simulink model "w3_warplab_trigger_proc"  (Simulink 7.7)
settings: Solver=ode45  StartTime=0.0  StopTime=60  RelTol=1e-3
InitFcn:
  | w3_warplab_trigger_proc_init
StartFcn:
  | w3_warplab_trigger_proc_init
undefined symbols (not defined in the file): gcbh, xlBlockLoadCallback, xlGetNormalizedPeriod
libraries: xbsIndex_r4 x1289, xbsEDKLib_r4 x1, simulink x1
(part 6 of 10)

== system w3_warplab_trigger_proc/Registers/Input Configuration Slice7 ==
  32b : Inport
  b30 : xbsIndex_r4/Slice  nbits=1  boolean_output=off  mode=Lower Bit Location + Width  bit1=0  base1=MSB of Input  bit0=30  base0=LSB of Input  dbl_ovrd=off  block_type=slice
  b31 : xbsIndex_r4/Slice  nbits=1  boolean_output=off  mode=Lower Bit Location + Width  bit1=0  base1=MSB of Input  bit0=31  base0=LSB of Input  dbl_ovrd=off  block_type=slice
  b[0:4] : xbsIndex_r4/Slice  nbits=5  boolean_output=off  mode=Lower Bit Location + Width  bit1=0  base1=MSB of Input  bit0=0  base0=LSB of Input  dbl_ovrd=off  block_type=slice
  Delay : Outport
  Debounce : Outport  Port=2
  Disable : Outport  Port=3
  wires:
  b31/1 -> Disable/1
  b30/1 -> Debounce/1
  b[0:4]/1 -> Delay/1
  32b/1 -> b[0:4]/1, b30/1, b31/1

== system w3_warplab_trigger_proc/Registers/Input Configuration Slice8 ==
  32b : Inport
  b29 : xbsIndex_r4/Slice  nbits=1  boolean_output=off  mode=Lower Bit Location + Width  bit1=0  base1=MSB of Input  bit0=29  base0=LSB of Input  dbl_ovrd=off  block_type=slice
  b30 : xbsIndex_r4/Slice  nbits=1  boolean_output=off  mode=Lower Bit Location + Width  bit1=0  base1=MSB of Input  bit0=30  base0=LSB of Input  dbl_ovrd=off  block_type=slice
  b31 : xbsIndex_r4/Slice  nbits=1  boolean_output=off  mode=Lower Bit Location + Width  bit1=0  base1=MSB of Input  bit0=31  base0=LSB of Input  dbl_ovrd=off  block_type=slice
  b[0:4] : xbsIndex_r4/Slice  nbits=5  boolean_output=off  mode=Lower Bit Location + Width  bit1=0  base1=MSB of Input  bit0=0  base0=LSB of Input  dbl_ovrd=off  block_type=slice
  Delay : Outport
  HW_SW_Sel : Outport  Port=2
  Debounce : Outport  Port=3
  Disable : Outport  Port=4
  wires:
  b31/1 -> Disable/1
  b30/1 -> Debounce/1
  b[0:4]/1 -> Delay/1
  32b/1 -> b[0:4]/1, b30/1, b31/1, b29/1
  b29/1 -> HW_SW_Sel/1

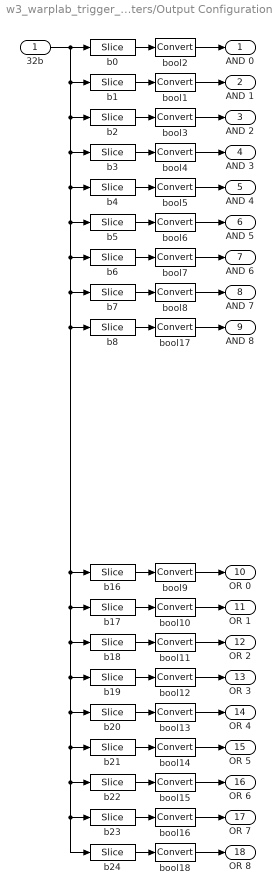
== system w3_warplab_trigger_proc/Registers/Output Configuration Slice ==
  32b : Inport
  b0 : xbsIndex_r4/Slice  nbits=1  boolean_output=off  mode=Lower Bit Location + Width  bit1=0  base1=MSB of Input  bit0=0  base0=LSB of Input  dbl_ovrd=off  block_type=slice
  b1 : xbsIndex_r4/Slice  nbits=1  boolean_output=off  mode=Lower Bit Location + Width  bit1=0  base1=MSB of Input  bit0=1  base0=LSB of Input  dbl_ovrd=off  block_type=slice
  b16 : xbsIndex_r4/Slice  nbits=1  boolean_output=off  mode=Lower Bit Location + Width  bit1=0  base1=MSB of Input  bit0=16  base0=LSB of Input  dbl_ovrd=off  block_type=slice
  b17 : xbsIndex_r4/Slice  nbits=1  boolean_output=off  mode=Lower Bit Location + Width  bit1=0  base1=MSB of Input  bit0=17  base0=LSB of Input  dbl_ovrd=off  block_type=slice
  b18 : xbsIndex_r4/Slice  nbits=1  boolean_output=off  mode=Lower Bit Location + Width  bit1=0  base1=MSB of Input  bit0=18  base0=LSB of Input  dbl_ovrd=off  block_type=slice
  b19 : xbsIndex_r4/Slice  nbits=1  boolean_output=off  mode=Lower Bit Location + Width  bit1=0  base1=MSB of Input  bit0=19  base0=LSB of Input  dbl_ovrd=off  block_type=slice
  b2 : xbsIndex_r4/Slice  nbits=1  boolean_output=off  mode=Lower Bit Location + Width  bit1=0  base1=MSB of Input  bit0=2  base0=LSB of Input  dbl_ovrd=off  block_type=slice
  b20 : xbsIndex_r4/Slice  nbits=1  boolean_output=off  mode=Lower Bit Location + Width  bit1=0  base1=MSB of Input  bit0=20  base0=LSB of Input  dbl_ovrd=off  block_type=slice
  b21 : xbsIndex_r4/Slice  nbits=1  boolean_output=off  mode=Lower Bit Location + Width  bit1=0  base1=MSB of Input  bit0=21  base0=LSB of Input  dbl_ovrd=off  block_type=slice
  b22 : xbsIndex_r4/Slice  nbits=1  boolean_output=off  mode=Lower Bit Location + Width  bit1=0  base1=MSB of Input  bit0=22  base0=LSB of Input  dbl_ovrd=off  block_type=slice
  b23 : xbsIndex_r4/Slice  nbits=1  boolean_output=off  mode=Lower Bit Location + Width  bit1=0  base1=MSB of Input  bit0=23  base0=LSB of Input  dbl_ovrd=off  block_type=slice
  b24 : xbsIndex_r4/Slice  nbits=1  boolean_output=off  mode=Lower Bit Location + Width  bit1=0  base1=MSB of Input  bit0=24  base0=LSB of Input  dbl_ovrd=off  block_type=slice
  b3 : xbsIndex_r4/Slice  nbits=1  boolean_output=off  mode=Lower Bit Location + Width  bit1=0  base1=MSB of Input  bit0=3  base0=LSB of Input  dbl_ovrd=off  block_type=slice
  b4 : xbsIndex_r4/Slice  nbits=1  boolean_output=off  mode=Lower Bit Location + Width  bit1=0  base1=MSB of Input  bit0=4  base0=LSB of Input  dbl_ovrd=off  block_type=slice
  b5 : xbsIndex_r4/Slice  nbits=1  boolean_output=off  mode=Lower Bit Location + Width  bit1=0  base1=MSB of Input  bit0=5  base0=LSB of Input  dbl_ovrd=off  block_type=slice
  b6 : xbsIndex_r4/Slice  nbits=1  boolean_output=off  mode=Lower Bit Location + Width  bit1=0  base1=MSB of Input  bit0=6  base0=LSB of Input  dbl_ovrd=off  block_type=slice
  b7 : xbsIndex_r4/Slice  nbits=1  boolean_output=off  mode=Lower Bit Location + Width  bit1=0  base1=MSB of Input  bit0=7  base0=LSB of Input  dbl_ovrd=off  block_type=slice
  b8 : xbsIndex_r4/Slice  nbits=1  boolean_output=off  mode=Lower Bit Location + Width  bit1=0  base1=MSB of Input  bit0=8  base0=LSB of Input  dbl_ovrd=off  block_type=slice
  bool{1..18} (18 alike) : xbsIndex_r4/Convert  gui_display_data_type=Boolean  arith_type=Boolean  n_bits=16  bin_pt=14  float_type=Single  exp_bits=8  fraction_bits=24  quantization=Truncate  overflow=Wrap  en=off  latency=0  dbl_ovrd=off  pipeline=off  block_type=convert
  AND 0 : Outport
  AND 1 : Outport  Port=2
  AND 2 : Outport  Port=3
  AND 3 : Outport  Port=4
  AND 4 : Outport  Port=5
  AND 5 : Outport  Port=6
  AND 6 : Outport  Port=7
  AND 7 : Outport  Port=8
  AND 8 : Outport  Port=9
  OR 0 : Outport  Port=10
  OR 1 : Outport  Port=11
  OR 2 : Outport  Port=12
  OR 3 : Outport  Port=13
  OR 4 : Outport  Port=14
  OR 5 : Outport  Port=15
  OR 6 : Outport  Port=16
  OR 7 : Outport  Port=17
  OR 8 : Outport  Port=18
  wires:
  32b/1 -> b0/1, b1/1, b2/1, b3/1, b4/1, b5/1, b6/1, b7/1, b16/1, b17/1, b18/1, b19/1, b20/1, b21/1, b22/1, b23/1, b24/1, b8/1
  b0/1 -> bool2/1
  b1/1 -> bool1/1
  b2/1 -> bool3/1
  b3/1 -> bool4/1
  b4/1 -> bool5/1
  b5/1 -> bool6/1
  b6/1 -> bool7/1
  b7/1 -> bool8/1
  b16/1 -> bool9/1
  b17/1 -> bool10/1
  b18/1 -> bool11/1
  b19/1 -> bool12/1
  b20/1 -> bool13/1
  b21/1 -> bool14/1
  b22/1 -> bool15/1
  b23/1 -> bool16/1
  bool2/1 -> AND 0/1
  bool1/1 -> AND 1/1
  bool3/1 -> AND 2/1
  bool4/1 -> AND 3/1
  bool5/1 -> AND 4/1
  bool6/1 -> AND 5/1
  bool7/1 -> AND 6/1
  bool8/1 -> AND 7/1
  bool9/1 -> OR 0/1
  bool10/1 -> OR 1/1
  bool11/1 -> OR 2/1
  bool12/1 -> OR 3/1
  bool13/1 -> OR 4/1
  bool14/1 -> OR 5/1
  bool15/1 -> OR 6/1
  bool16/1 -> OR 7/1
  b8/1 -> bool17/1
  bool17/1 -> AND 8/1
  b24/1 -> bool18/1
  bool18/1 -> OR 8/1

== system w3_warplab_trigger_proc/Registers/Output Configuration Slice1 ==
  32b : Inport
  b30 : xbsIndex_r4/Slice  nbits=1  boolean_output=off  mode=Lower Bit Location + Width  bit1=0  base1=MSB of Input  bit0=30  base0=LSB of Input  dbl_ovrd=off  block_type=slice
  b31 : xbsIndex_r4/Slice  nbits=1  boolean_output=off  mode=Lower Bit Location + Width  bit1=0  base1=MSB of Input  bit0=31  base0=LSB of Input  dbl_ovrd=off  block_type=slice
  b[0:15] : xbsIndex_r4/Slice  nbits=16  boolean_output=off  mode=Lower Bit Location + Width  bit1=0  base1=MSB of Input  bit0=0  base0=LSB of Input  dbl_ovrd=off  block_type=slice
  bool1 : xbsIndex_r4/Convert  gui_display_data_type=Boolean  arith_type=Boolean  n_bits=16  bin_pt=14  float_type=Single  exp_bits=8  fraction_bits=24  quantization=Truncate  overflow=Wrap  en=off  latency=0  dbl_ovrd=off  pipeline=off  block_type=convert
  bool17 : xbsIndex_r4/Convert  gui_display_data_type=Boolean  arith_type=Boolean  n_bits=16  bin_pt=14  float_type=Single  exp_bits=8  fraction_bits=24  quantization=Truncate  overflow=Wrap  en=off  latency=0  dbl_ovrd=off  pipeline=off  block_type=convert
  DELAY : Outport
  BYPASS : Outport  Port=2
  DISABLE : Outport  Port=3
  wires:
  32b/1 -> b[0:15]/1, b31/1, b30/1
  b31/1 -> bool17/1
  bool17/1 -> DISABLE/1
  b[0:15]/1 -> DELAY/1
  b30/1 -> bool1/1
  bool1/1 -> BYPASS/1

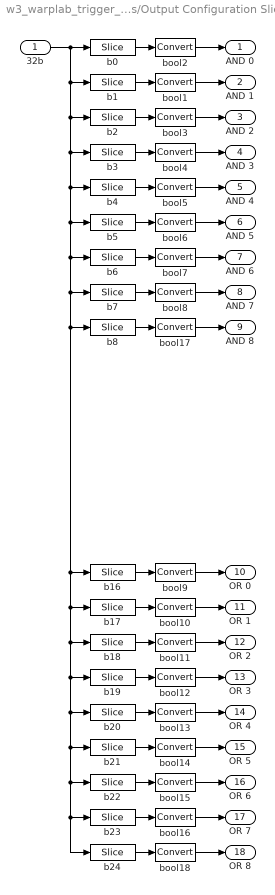
== system w3_warplab_trigger_proc/Registers/Output Configuration Slice12 ==
  32b : Inport
  b0 : xbsIndex_r4/Slice  nbits=1  boolean_output=off  mode=Lower Bit Location + Width  bit1=0  base1=MSB of Input  bit0=0  base0=LSB of Input  dbl_ovrd=off  block_type=slice
  b1 : xbsIndex_r4/Slice  nbits=1  boolean_output=off  mode=Lower Bit Location + Width  bit1=0  base1=MSB of Input  bit0=1  base0=LSB of Input  dbl_ovrd=off  block_type=slice
  b16 : xbsIndex_r4/Slice  nbits=1  boolean_output=off  mode=Lower Bit Location + Width  bit1=0  base1=MSB of Input  bit0=16  base0=LSB of Input  dbl_ovrd=off  block_type=slice
  b17 : xbsIndex_r4/Slice  nbits=1  boolean_output=off  mode=Lower Bit Location + Width  bit1=0  base1=MSB of Input  bit0=17  base0=LSB of Input  dbl_ovrd=off  block_type=slice
  b18 : xbsIndex_r4/Slice  nbits=1  boolean_output=off  mode=Lower Bit Location + Width  bit1=0  base1=MSB of Input  bit0=18  base0=LSB of Input  dbl_ovrd=off  block_type=slice
  b19 : xbsIndex_r4/Slice  nbits=1  boolean_output=off  mode=Lower Bit Location + Width  bit1=0  base1=MSB of Input  bit0=19  base0=LSB of Input  dbl_ovrd=off  block_type=slice
  b2 : xbsIndex_r4/Slice  nbits=1  boolean_output=off  mode=Lower Bit Location + Width  bit1=0  base1=MSB of Input  bit0=2  base0=LSB of Input  dbl_ovrd=off  block_type=slice
  b20 : xbsIndex_r4/Slice  nbits=1  boolean_output=off  mode=Lower Bit Location + Width  bit1=0  base1=MSB of Input  bit0=20  base0=LSB of Input  dbl_ovrd=off  block_type=slice
  b21 : xbsIndex_r4/Slice  nbits=1  boolean_output=off  mode=Lower Bit Location + Width  bit1=0  base1=MSB of Input  bit0=21  base0=LSB of Input  dbl_ovrd=off  block_type=slice
  b22 : xbsIndex_r4/Slice  nbits=1  boolean_output=off  mode=Lower Bit Location + Width  bit1=0  base1=MSB of Input  bit0=22  base0=LSB of Input  dbl_ovrd=off  block_type=slice
  b23 : xbsIndex_r4/Slice  nbits=1  boolean_output=off  mode=Lower Bit Location + Width  bit1=0  base1=MSB of Input  bit0=23  base0=LSB of Input  dbl_ovrd=off  block_type=slice
  b24 : xbsIndex_r4/Slice  nbits=1  boolean_output=off  mode=Lower Bit Location + Width  bit1=0  base1=MSB of Input  bit0=24  base0=LSB of Input  dbl_ovrd=off  block_type=slice
  b3 : xbsIndex_r4/Slice  nbits=1  boolean_output=off  mode=Lower Bit Location + Width  bit1=0  base1=MSB of Input  bit0=3  base0=LSB of Input  dbl_ovrd=off  block_type=slice
  b4 : xbsIndex_r4/Slice  nbits=1  boolean_output=off  mode=Lower Bit Location + Width  bit1=0  base1=MSB of Input  bit0=4  base0=LSB of Input  dbl_ovrd=off  block_type=slice
  b5 : xbsIndex_r4/Slice  nbits=1  boolean_output=off  mode=Lower Bit Location + Width  bit1=0  base1=MSB of Input  bit0=5  base0=LSB of Input  dbl_ovrd=off  block_type=slice
  b6 : xbsIndex_r4/Slice  nbits=1  boolean_output=off  mode=Lower Bit Location + Width  bit1=0  base1=MSB of Input  bit0=6  base0=LSB of Input  dbl_ovrd=off  block_type=slice
  b7 : xbsIndex_r4/Slice  nbits=1  boolean_output=off  mode=Lower Bit Location + Width  bit1=0  base1=MSB of Input  bit0=7  base0=LSB of Input  dbl_ovrd=off  block_type=slice
  b8 : xbsIndex_r4/Slice  nbits=1  boolean_output=off  mode=Lower Bit Location + Width  bit1=0  base1=MSB of Input  bit0=8  base0=LSB of Input  dbl_ovrd=off  block_type=slice
  bool{1..18} (18 alike) : xbsIndex_r4/Convert  gui_display_data_type=Boolean  arith_type=Boolean  n_bits=16  bin_pt=14  float_type=Single  exp_bits=8  fraction_bits=24  quantization=Truncate  overflow=Wrap  en=off  latency=0  dbl_ovrd=off  pipeline=off  block_type=convert
  AND 0 : Outport
  AND 1 : Outport  Port=2
  AND 2 : Outport  Port=3
  AND 3 : Outport  Port=4
  AND 4 : Outport  Port=5
  AND 5 : Outport  Port=6
  AND 6 : Outport  Port=7
  AND 7 : Outport  Port=8
  AND 8 : Outport  Port=9
  OR 0 : Outport  Port=10
  OR 1 : Outport  Port=11
  OR 2 : Outport  Port=12
  OR 3 : Outport  Port=13
  OR 4 : Outport  Port=14
  OR 5 : Outport  Port=15
  OR 6 : Outport  Port=16
  OR 7 : Outport  Port=17
  OR 8 : Outport  Port=18
  wires:
  32b/1 -> b0/1, b1/1, b2/1, b3/1, b4/1, b5/1, b6/1, b7/1, b16/1, b17/1, b18/1, b19/1, b20/1, b21/1, b22/1, b23/1, b24/1, b8/1
  b0/1 -> bool2/1
  b1/1 -> bool1/1
  b2/1 -> bool3/1
  b3/1 -> bool4/1
  b4/1 -> bool5/1
  b5/1 -> bool6/1
  b6/1 -> bool7/1
  b7/1 -> bool8/1
  b16/1 -> bool9/1
  b17/1 -> bool10/1
  b18/1 -> bool11/1
  b19/1 -> bool12/1
  b20/1 -> bool13/1
  b21/1 -> bool14/1
  b22/1 -> bool15/1
  b23/1 -> bool16/1
  bool2/1 -> AND 0/1
  bool1/1 -> AND 1/1
  bool3/1 -> AND 2/1
  bool4/1 -> AND 3/1
  bool5/1 -> AND 4/1
  bool6/1 -> AND 5/1
  bool7/1 -> AND 6/1
  bool8/1 -> AND 7/1
  bool9/1 -> OR 0/1
  bool10/1 -> OR 1/1
  bool11/1 -> OR 2/1
  bool12/1 -> OR 3/1
  bool13/1 -> OR 4/1
  bool14/1 -> OR 5/1
  bool15/1 -> OR 6/1
  bool16/1 -> OR 7/1
  b8/1 -> bool17/1
  bool17/1 -> AND 8/1
  b24/1 -> bool18/1
  bool18/1 -> OR 8/1

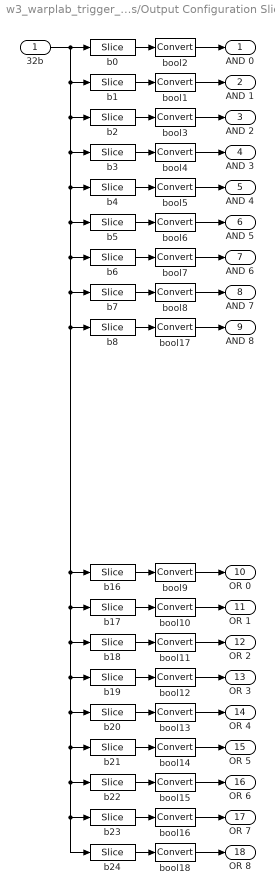
== system w3_warplab_trigger_proc/Registers/Output Configuration Slice14 ==
  32b : Inport
  b0 : xbsIndex_r4/Slice  nbits=1  boolean_output=off  mode=Lower Bit Location + Width  bit1=0  base1=MSB of Input  bit0=0  base0=LSB of Input  dbl_ovrd=off  block_type=slice
  b1 : xbsIndex_r4/Slice  nbits=1  boolean_output=off  mode=Lower Bit Location + Width  bit1=0  base1=MSB of Input  bit0=1  base0=LSB of Input  dbl_ovrd=off  block_type=slice
  b16 : xbsIndex_r4/Slice  nbits=1  boolean_output=off  mode=Lower Bit Location + Width  bit1=0  base1=MSB of Input  bit0=16  base0=LSB of Input  dbl_ovrd=off  block_type=slice
  b17 : xbsIndex_r4/Slice  nbits=1  boolean_output=off  mode=Lower Bit Location + Width  bit1=0  base1=MSB of Input  bit0=17  base0=LSB of Input  dbl_ovrd=off  block_type=slice
  b18 : xbsIndex_r4/Slice  nbits=1  boolean_output=off  mode=Lower Bit Location + Width  bit1=0  base1=MSB of Input  bit0=18  base0=LSB of Input  dbl_ovrd=off  block_type=slice
  b19 : xbsIndex_r4/Slice  nbits=1  boolean_output=off  mode=Lower Bit Location + Width  bit1=0  base1=MSB of Input  bit0=19  base0=LSB of Input  dbl_ovrd=off  block_type=slice
  b2 : xbsIndex_r4/Slice  nbits=1  boolean_output=off  mode=Lower Bit Location + Width  bit1=0  base1=MSB of Input  bit0=2  base0=LSB of Input  dbl_ovrd=off  block_type=slice
  b20 : xbsIndex_r4/Slice  nbits=1  boolean_output=off  mode=Lower Bit Location + Width  bit1=0  base1=MSB of Input  bit0=20  base0=LSB of Input  dbl_ovrd=off  block_type=slice
  b21 : xbsIndex_r4/Slice  nbits=1  boolean_output=off  mode=Lower Bit Location + Width  bit1=0  base1=MSB of Input  bit0=21  base0=LSB of Input  dbl_ovrd=off  block_type=slice
  b22 : xbsIndex_r4/Slice  nbits=1  boolean_output=off  mode=Lower Bit Location + Width  bit1=0  base1=MSB of Input  bit0=22  base0=LSB of Input  dbl_ovrd=off  block_type=slice
  b23 : xbsIndex_r4/Slice  nbits=1  boolean_output=off  mode=Lower Bit Location + Width  bit1=0  base1=MSB of Input  bit0=23  base0=LSB of Input  dbl_ovrd=off  block_type=slice
  b24 : xbsIndex_r4/Slice  nbits=1  boolean_output=off  mode=Lower Bit Location + Width  bit1=0  base1=MSB of Input  bit0=24  base0=LSB of Input  dbl_ovrd=off  block_type=slice
  b3 : xbsIndex_r4/Slice  nbits=1  boolean_output=off  mode=Lower Bit Location + Width  bit1=0  base1=MSB of Input  bit0=3  base0=LSB of Input  dbl_ovrd=off  block_type=slice
  b4 : xbsIndex_r4/Slice  nbits=1  boolean_output=off  mode=Lower Bit Location + Width  bit1=0  base1=MSB of Input  bit0=4  base0=LSB of Input  dbl_ovrd=off  block_type=slice
  b5 : xbsIndex_r4/Slice  nbits=1  boolean_output=off  mode=Lower Bit Location + Width  bit1=0  base1=MSB of Input  bit0=5  base0=LSB of Input  dbl_ovrd=off  block_type=slice
  b6 : xbsIndex_r4/Slice  nbits=1  boolean_output=off  mode=Lower Bit Location + Width  bit1=0  base1=MSB of Input  bit0=6  base0=LSB of Input  dbl_ovrd=off  block_type=slice
  b7 : xbsIndex_r4/Slice  nbits=1  boolean_output=off  mode=Lower Bit Location + Width  bit1=0  base1=MSB of Input  bit0=7  base0=LSB of Input  dbl_ovrd=off  block_type=slice
  b8 : xbsIndex_r4/Slice  nbits=1  boolean_output=off  mode=Lower Bit Location + Width  bit1=0  base1=MSB of Input  bit0=8  base0=LSB of Input  dbl_ovrd=off  block_type=slice
  bool{1..18} (18 alike) : xbsIndex_r4/Convert  gui_display_data_type=Boolean  arith_type=Boolean  n_bits=16  bin_pt=14  float_type=Single  exp_bits=8  fraction_bits=24  quantization=Truncate  overflow=Wrap  en=off  latency=0  dbl_ovrd=off  pipeline=off  block_type=convert
  AND 0 : Outport
  AND 1 : Outport  Port=2
  AND 2 : Outport  Port=3
  AND 3 : Outport  Port=4
  AND 4 : Outport  Port=5
  AND 5 : Outport  Port=6
  AND 6 : Outport  Port=7
  AND 7 : Outport  Port=8
  AND 8 : Outport  Port=9
  OR 0 : Outport  Port=10
  OR 1 : Outport  Port=11
  OR 2 : Outport  Port=12
  OR 3 : Outport  Port=13
  OR 4 : Outport  Port=14
  OR 5 : Outport  Port=15
  OR 6 : Outport  Port=16
  OR 7 : Outport  Port=17
  OR 8 : Outport  Port=18
  wires:
  32b/1 -> b0/1, b1/1, b2/1, b3/1, b4/1, b5/1, b6/1, b7/1, b16/1, b17/1, b18/1, b19/1, b20/1, b21/1, b22/1, b23/1, b24/1, b8/1
  b0/1 -> bool2/1
  b1/1 -> bool1/1
  b2/1 -> bool3/1
  b3/1 -> bool4/1
  b4/1 -> bool5/1
  b5/1 -> bool6/1
  b6/1 -> bool7/1
  b7/1 -> bool8/1
  b16/1 -> bool9/1
  b17/1 -> bool10/1
  b18/1 -> bool11/1
  b19/1 -> bool12/1
  b20/1 -> bool13/1
  b21/1 -> bool14/1
  b22/1 -> bool15/1
  b23/1 -> bool16/1
  bool2/1 -> AND 0/1
  bool1/1 -> AND 1/1
  bool3/1 -> AND 2/1
  bool4/1 -> AND 3/1
  bool5/1 -> AND 4/1
  bool6/1 -> AND 5/1
  bool7/1 -> AND 6/1
  bool8/1 -> AND 7/1
  bool9/1 -> OR 0/1
  bool10/1 -> OR 1/1
  bool11/1 -> OR 2/1
  bool12/1 -> OR 3/1
  bool13/1 -> OR 4/1
  bool14/1 -> OR 5/1
  bool15/1 -> OR 6/1
  bool16/1 -> OR 7/1
  b8/1 -> bool17/1
  bool17/1 -> AND 8/1
  b24/1 -> bool18/1
  bool18/1 -> OR 8/1

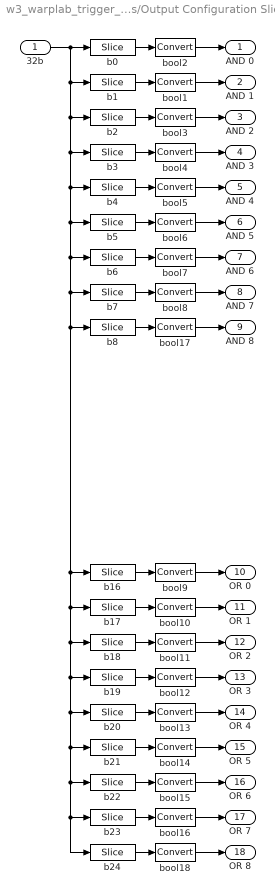
== system w3_warplab_trigger_proc/Registers/Output Configuration Slice16 ==
  32b : Inport
  b0 : xbsIndex_r4/Slice  nbits=1  boolean_output=off  mode=Lower Bit Location + Width  bit1=0  base1=MSB of Input  bit0=0  base0=LSB of Input  dbl_ovrd=off  block_type=slice
  b1 : xbsIndex_r4/Slice  nbits=1  boolean_output=off  mode=Lower Bit Location + Width  bit1=0  base1=MSB of Input  bit0=1  base0=LSB of Input  dbl_ovrd=off  block_type=slice
  b16 : xbsIndex_r4/Slice  nbits=1  boolean_output=off  mode=Lower Bit Location + Width  bit1=0  base1=MSB of Input  bit0=16  base0=LSB of Input  dbl_ovrd=off  block_type=slice
  b17 : xbsIndex_r4/Slice  nbits=1  boolean_output=off  mode=Lower Bit Location + Width  bit1=0  base1=MSB of Input  bit0=17  base0=LSB of Input  dbl_ovrd=off  block_type=slice
  b18 : xbsIndex_r4/Slice  nbits=1  boolean_output=off  mode=Lower Bit Location + Width  bit1=0  base1=MSB of Input  bit0=18  base0=LSB of Input  dbl_ovrd=off  block_type=slice
  b19 : xbsIndex_r4/Slice  nbits=1  boolean_output=off  mode=Lower Bit Location + Width  bit1=0  base1=MSB of Input  bit0=19  base0=LSB of Input  dbl_ovrd=off  block_type=slice
  b2 : xbsIndex_r4/Slice  nbits=1  boolean_output=off  mode=Lower Bit Location + Width  bit1=0  base1=MSB of Input  bit0=2  base0=LSB of Input  dbl_ovrd=off  block_type=slice
  b20 : xbsIndex_r4/Slice  nbits=1  boolean_output=off  mode=Lower Bit Location + Width  bit1=0  base1=MSB of Input  bit0=20  base0=LSB of Input  dbl_ovrd=off  block_type=slice
  b21 : xbsIndex_r4/Slice  nbits=1  boolean_output=off  mode=Lower Bit Location + Width  bit1=0  base1=MSB of Input  bit0=21  base0=LSB of Input  dbl_ovrd=off  block_type=slice
  b22 : xbsIndex_r4/Slice  nbits=1  boolean_output=off  mode=Lower Bit Location + Width  bit1=0  base1=MSB of Input  bit0=22  base0=LSB of Input  dbl_ovrd=off  block_type=slice
  b23 : xbsIndex_r4/Slice  nbits=1  boolean_output=off  mode=Lower Bit Location + Width  bit1=0  base1=MSB of Input  bit0=23  base0=LSB of Input  dbl_ovrd=off  block_type=slice
  b24 : xbsIndex_r4/Slice  nbits=1  boolean_output=off  mode=Lower Bit Location + Width  bit1=0  base1=MSB of Input  bit0=24  base0=LSB of Input  dbl_ovrd=off  block_type=slice
  b3 : xbsIndex_r4/Slice  nbits=1  boolean_output=off  mode=Lower Bit Location + Width  bit1=0  base1=MSB of Input  bit0=3  base0=LSB of Input  dbl_ovrd=off  block_type=slice
  b4 : xbsIndex_r4/Slice  nbits=1  boolean_output=off  mode=Lower Bit Location + Width  bit1=0  base1=MSB of Input  bit0=4  base0=LSB of Input  dbl_ovrd=off  block_type=slice
  b5 : xbsIndex_r4/Slice  nbits=1  boolean_output=off  mode=Lower Bit Location + Width  bit1=0  base1=MSB of Input  bit0=5  base0=LSB of Input  dbl_ovrd=off  block_type=slice
  b6 : xbsIndex_r4/Slice  nbits=1  boolean_output=off  mode=Lower Bit Location + Width  bit1=0  base1=MSB of Input  bit0=6  base0=LSB of Input  dbl_ovrd=off  block_type=slice
  b7 : xbsIndex_r4/Slice  nbits=1  boolean_output=off  mode=Lower Bit Location + Width  bit1=0  base1=MSB of Input  bit0=7  base0=LSB of Input  dbl_ovrd=off  block_type=slice
  b8 : xbsIndex_r4/Slice  nbits=1  boolean_output=off  mode=Lower Bit Location + Width  bit1=0  base1=MSB of Input  bit0=8  base0=LSB of Input  dbl_ovrd=off  block_type=slice
  bool{1..18} (18 alike) : xbsIndex_r4/Convert  gui_display_data_type=Boolean  arith_type=Boolean  n_bits=16  bin_pt=14  float_type=Single  exp_bits=8  fraction_bits=24  quantization=Truncate  overflow=Wrap  en=off  latency=0  dbl_ovrd=off  pipeline=off  block_type=convert
  AND 0 : Outport
  AND 1 : Outport  Port=2
  AND 2 : Outport  Port=3
  AND 3 : Outport  Port=4
  AND 4 : Outport  Port=5
  AND 5 : Outport  Port=6
  AND 6 : Outport  Port=7
  AND 7 : Outport  Port=8
  AND 8 : Outport  Port=9
  OR 0 : Outport  Port=10
  OR 1 : Outport  Port=11
  OR 2 : Outport  Port=12
  OR 3 : Outport  Port=13
  OR 4 : Outport  Port=14
  OR 5 : Outport  Port=15
  OR 6 : Outport  Port=16
  OR 7 : Outport  Port=17
  OR 8 : Outport  Port=18
  wires:
  32b/1 -> b0/1, b1/1, b2/1, b3/1, b4/1, b5/1, b6/1, b7/1, b16/1, b17/1, b18/1, b19/1, b20/1, b21/1, b22/1, b23/1, b24/1, b8/1
  b0/1 -> bool2/1
  b1/1 -> bool1/1
  b2/1 -> bool3/1
  b3/1 -> bool4/1
  b4/1 -> bool5/1
  b5/1 -> bool6/1
  b6/1 -> bool7/1
  b7/1 -> bool8/1
  b16/1 -> bool9/1
  b17/1 -> bool10/1
  b18/1 -> bool11/1
  b19/1 -> bool12/1
  b20/1 -> bool13/1
  b21/1 -> bool14/1
  b22/1 -> bool15/1
  b23/1 -> bool16/1
  bool2/1 -> AND 0/1
  bool1/1 -> AND 1/1
  bool3/1 -> AND 2/1
  bool4/1 -> AND 3/1
  bool5/1 -> AND 4/1
  bool6/1 -> AND 5/1
  bool7/1 -> AND 6/1
  bool8/1 -> AND 7/1
  bool9/1 -> OR 0/1
  bool10/1 -> OR 1/1
  bool11/1 -> OR 2/1
  bool12/1 -> OR 3/1
  bool13/1 -> OR 4/1
  bool14/1 -> OR 5/1
  bool15/1 -> OR 6/1
  bool16/1 -> OR 7/1
  b8/1 -> bool17/1
  bool17/1 -> AND 8/1
  b24/1 -> bool18/1
  bool18/1 -> OR 8/1

== system w3_warplab_trigger_proc/Registers/Output Configuration Slice2 ==
  32b : Inport
  b30 : xbsIndex_r4/Slice  nbits=1  boolean_output=off  mode=Lower Bit Location + Width  bit1=0  base1=MSB of Input  bit0=30  base0=LSB of Input  dbl_ovrd=off  block_type=slice
  b31 : xbsIndex_r4/Slice  nbits=1  boolean_output=off  mode=Lower Bit Location + Width  bit1=0  base1=MSB of Input  bit0=31  base0=LSB of Input  dbl_ovrd=off  block_type=slice
  b[0:15] : xbsIndex_r4/Slice  nbits=16  boolean_output=off  mode=Lower Bit Location + Width  bit1=0  base1=MSB of Input  bit0=0  base0=LSB of Input  dbl_ovrd=off  block_type=slice
  bool1 : xbsIndex_r4/Convert  gui_display_data_type=Boolean  arith_type=Boolean  n_bits=16  bin_pt=14  float_type=Single  exp_bits=8  fraction_bits=24  quantization=Truncate  overflow=Wrap  en=off  latency=0  dbl_ovrd=off  pipeline=off  block_type=convert
  bool17 : xbsIndex_r4/Convert  gui_display_data_type=Boolean  arith_type=Boolean  n_bits=16  bin_pt=14  float_type=Single  exp_bits=8  fraction_bits=24  quantization=Truncate  overflow=Wrap  en=off  latency=0  dbl_ovrd=off  pipeline=off  block_type=convert
  DELAY : Outport
  BYPASS : Outport  Port=2
  DISABLE : Outport  Port=3
  wires:
  32b/1 -> b[0:15]/1, b31/1, b30/1
  b31/1 -> bool17/1
  bool17/1 -> DISABLE/1
  b[0:15]/1 -> DELAY/1
  b30/1 -> bool1/1
  bool1/1 -> BYPASS/1

== system w3_warplab_trigger_proc/Registers/Output Configuration Slice3 ==
  32b : Inport
  b30 : xbsIndex_r4/Slice  nbits=1  boolean_output=off  mode=Lower Bit Location + Width  bit1=0  base1=MSB of Input  bit0=30  base0=LSB of Input  dbl_ovrd=off  block_type=slice
  b31 : xbsIndex_r4/Slice  nbits=1  boolean_output=off  mode=Lower Bit Location + Width  bit1=0  base1=MSB of Input  bit0=31  base0=LSB of Input  dbl_ovrd=off  block_type=slice
  b[0:15] : xbsIndex_r4/Slice  nbits=16  boolean_output=off  mode=Lower Bit Location + Width  bit1=0  base1=MSB of Input  bit0=0  base0=LSB of Input  dbl_ovrd=off  block_type=slice
  bool1 : xbsIndex_r4/Convert  gui_display_data_type=Boolean  arith_type=Boolean  n_bits=16  bin_pt=14  float_type=Single  exp_bits=8  fraction_bits=24  quantization=Truncate  overflow=Wrap  en=off  latency=0  dbl_ovrd=off  pipeline=off  block_type=convert
  bool17 : xbsIndex_r4/Convert  gui_display_data_type=Boolean  arith_type=Boolean  n_bits=16  bin_pt=14  float_type=Single  exp_bits=8  fraction_bits=24  quantization=Truncate  overflow=Wrap  en=off  latency=0  dbl_ovrd=off  pipeline=off  block_type=convert
  DELAY : Outport
  BYPASS : Outport  Port=2
  DISABLE : Outport  Port=3
  wires:
  32b/1 -> b[0:15]/1, b31/1, b30/1
  b31/1 -> bool17/1
  bool17/1 -> DISABLE/1
  b[0:15]/1 -> DELAY/1
  b30/1 -> bool1/1
  bool1/1 -> BYPASS/1

== system w3_warplab_trigger_proc/Registers/Output Configuration Slice4 ==
  32b : Inport
  b30 : xbsIndex_r4/Slice  nbits=1  boolean_output=off  mode=Lower Bit Location + Width  bit1=0  base1=MSB of Input  bit0=30  base0=LSB of Input  dbl_ovrd=off  block_type=slice
  b31 : xbsIndex_r4/Slice  nbits=1  boolean_output=off  mode=Lower Bit Location + Width  bit1=0  base1=MSB of Input  bit0=31  base0=LSB of Input  dbl_ovrd=off  block_type=slice
  b[0:15] : xbsIndex_r4/Slice  nbits=16  boolean_output=off  mode=Lower Bit Location + Width  bit1=0  base1=MSB of Input  bit0=0  base0=LSB of Input  dbl_ovrd=off  block_type=slice
  bool1 : xbsIndex_r4/Convert  gui_display_data_type=Boolean  arith_type=Boolean  n_bits=16  bin_pt=14  float_type=Single  exp_bits=8  fraction_bits=24  quantization=Truncate  overflow=Wrap  en=off  latency=0  dbl_ovrd=off  pipeline=off  block_type=convert
  bool17 : xbsIndex_r4/Convert  gui_display_data_type=Boolean  arith_type=Boolean  n_bits=16  bin_pt=14  float_type=Single  exp_bits=8  fraction_bits=24  quantization=Truncate  overflow=Wrap  en=off  latency=0  dbl_ovrd=off  pipeline=off  block_type=convert
  DELAY : Outport
  BYPASS : Outport  Port=2
  DISABLE : Outport  Port=3
  wires:
  32b/1 -> b[0:15]/1, b31/1, b30/1
  b31/1 -> bool17/1
  bool17/1 -> DISABLE/1
  b[0:15]/1 -> DELAY/1
  b30/1 -> bool1/1
  bool1/1 -> BYPASS/1

== system w3_warplab_trigger_proc/Registers/Output Configuration Slice5 ==
  32b : Inport
  b30 : xbsIndex_r4/Slice  nbits=1  boolean_output=off  mode=Lower Bit Location + Width  bit1=0  base1=MSB of Input  bit0=30  base0=LSB of Input  dbl_ovrd=off  block_type=slice
  b31 : xbsIndex_r4/Slice  nbits=1  boolean_output=off  mode=Lower Bit Location + Width  bit1=0  base1=MSB of Input  bit0=31  base0=LSB of Input  dbl_ovrd=off  block_type=slice
  b[0:15] : xbsIndex_r4/Slice  nbits=16  boolean_output=off  mode=Lower Bit Location + Width  bit1=0  base1=MSB of Input  bit0=0  base0=LSB of Input  dbl_ovrd=off  block_type=slice
  bool1 : xbsIndex_r4/Convert  gui_display_data_type=Boolean  arith_type=Boolean  n_bits=16  bin_pt=14  float_type=Single  exp_bits=8  fraction_bits=24  quantization=Truncate  overflow=Wrap  en=off  latency=0  dbl_ovrd=off  pipeline=off  block_type=convert
  bool17 : xbsIndex_r4/Convert  gui_display_data_type=Boolean  arith_type=Boolean  n_bits=16  bin_pt=14  float_type=Single  exp_bits=8  fraction_bits=24  quantization=Truncate  overflow=Wrap  en=off  latency=0  dbl_ovrd=off  pipeline=off  block_type=convert
  DELAY : Outport
  BYPASS : Outport  Port=2
  DISABLE : Outport  Port=3
  wires:
  32b/1 -> b[0:15]/1, b31/1, b30/1
  b31/1 -> bool17/1
  bool17/1 -> DISABLE/1
  b[0:15]/1 -> DELAY/1
  b30/1 -> bool1/1
  bool1/1 -> BYPASS/1

== system w3_warplab_trigger_proc/Registers/Output Configuration Slice6 ==
  32b : Inport
  b30 : xbsIndex_r4/Slice  nbits=1  boolean_output=off  mode=Lower Bit Location + Width  bit1=0  base1=MSB of Input  bit0=30  base0=LSB of Input  dbl_ovrd=off  block_type=slice
  b31 : xbsIndex_r4/Slice  nbits=1  boolean_output=off  mode=Lower Bit Location + Width  bit1=0  base1=MSB of Input  bit0=31  base0=LSB of Input  dbl_ovrd=off  block_type=slice
  b[0:15] : xbsIndex_r4/Slice  nbits=16  boolean_output=off  mode=Lower Bit Location + Width  bit1=0  base1=MSB of Input  bit0=0  base0=LSB of Input  dbl_ovrd=off  block_type=slice
  bool1 : xbsIndex_r4/Convert  gui_display_data_type=Boolean  arith_type=Boolean  n_bits=16  bin_pt=14  float_type=Single  exp_bits=8  fraction_bits=24  quantization=Truncate  overflow=Wrap  en=off  latency=0  dbl_ovrd=off  pipeline=off  block_type=convert
  bool17 : xbsIndex_r4/Convert  gui_display_data_type=Boolean  arith_type=Boolean  n_bits=16  bin_pt=14  float_type=Single  exp_bits=8  fraction_bits=24  quantization=Truncate  overflow=Wrap  en=off  latency=0  dbl_ovrd=off  pipeline=off  block_type=convert
  DELAY : Outport
  BYPASS : Outport  Port=2
  DISABLE : Outport  Port=3
  wires:
  32b/1 -> b[0:15]/1, b31/1, b30/1
  b31/1 -> bool17/1
  bool17/1 -> DISABLE/1
  b[0:15]/1 -> DELAY/1
  b30/1 -> bool1/1
  bool1/1 -> BYPASS/1

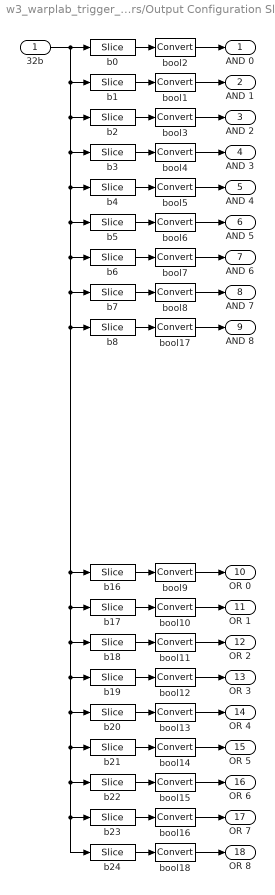
== system w3_warplab_trigger_proc/Registers/Output Configuration Slice7 ==
  32b : Inport
  b0 : xbsIndex_r4/Slice  nbits=1  boolean_output=off  mode=Lower Bit Location + Width  bit1=0  base1=MSB of Input  bit0=0  base0=LSB of Input  dbl_ovrd=off  block_type=slice
  b1 : xbsIndex_r4/Slice  nbits=1  boolean_output=off  mode=Lower Bit Location + Width  bit1=0  base1=MSB of Input  bit0=1  base0=LSB of Input  dbl_ovrd=off  block_type=slice
  b16 : xbsIndex_r4/Slice  nbits=1  boolean_output=off  mode=Lower Bit Location + Width  bit1=0  base1=MSB of Input  bit0=16  base0=LSB of Input  dbl_ovrd=off  block_type=slice
  b17 : xbsIndex_r4/Slice  nbits=1  boolean_output=off  mode=Lower Bit Location + Width  bit1=0  base1=MSB of Input  bit0=17  base0=LSB of Input  dbl_ovrd=off  block_type=slice
  b18 : xbsIndex_r4/Slice  nbits=1  boolean_output=off  mode=Lower Bit Location + Width  bit1=0  base1=MSB of Input  bit0=18  base0=LSB of Input  dbl_ovrd=off  block_type=slice
  b19 : xbsIndex_r4/Slice  nbits=1  boolean_output=off  mode=Lower Bit Location + Width  bit1=0  base1=MSB of Input  bit0=19  base0=LSB of Input  dbl_ovrd=off  block_type=slice
  b2 : xbsIndex_r4/Slice  nbits=1  boolean_output=off  mode=Lower Bit Location + Width  bit1=0  base1=MSB of Input  bit0=2  base0=LSB of Input  dbl_ovrd=off  block_type=slice
  b20 : xbsIndex_r4/Slice  nbits=1  boolean_output=off  mode=Lower Bit Location + Width  bit1=0  base1=MSB of Input  bit0=20  base0=LSB of Input  dbl_ovrd=off  block_type=slice
  b21 : xbsIndex_r4/Slice  nbits=1  boolean_output=off  mode=Lower Bit Location + Width  bit1=0  base1=MSB of Input  bit0=21  base0=LSB of Input  dbl_ovrd=off  block_type=slice
  b22 : xbsIndex_r4/Slice  nbits=1  boolean_output=off  mode=Lower Bit Location + Width  bit1=0  base1=MSB of Input  bit0=22  base0=LSB of Input  dbl_ovrd=off  block_type=slice
  b23 : xbsIndex_r4/Slice  nbits=1  boolean_output=off  mode=Lower Bit Location + Width  bit1=0  base1=MSB of Input  bit0=23  base0=LSB of Input  dbl_ovrd=off  block_type=slice
  b24 : xbsIndex_r4/Slice  nbits=1  boolean_output=off  mode=Lower Bit Location + Width  bit1=0  base1=MSB of Input  bit0=24  base0=LSB of Input  dbl_ovrd=off  block_type=slice
  b3 : xbsIndex_r4/Slice  nbits=1  boolean_output=off  mode=Lower Bit Location + Width  bit1=0  base1=MSB of Input  bit0=3  base0=LSB of Input  dbl_ovrd=off  block_type=slice
  b4 : xbsIndex_r4/Slice  nbits=1  boolean_output=off  mode=Lower Bit Location + Width  bit1=0  base1=MSB of Input  bit0=4  base0=LSB of Input  dbl_ovrd=off  block_type=slice
  b5 : xbsIndex_r4/Slice  nbits=1  boolean_output=off  mode=Lower Bit Location + Width  bit1=0  base1=MSB of Input  bit0=5  base0=LSB of Input  dbl_ovrd=off  block_type=slice
  b6 : xbsIndex_r4/Slice  nbits=1  boolean_output=off  mode=Lower Bit Location + Width  bit1=0  base1=MSB of Input  bit0=6  base0=LSB of Input  dbl_ovrd=off  block_type=slice
  b7 : xbsIndex_r4/Slice  nbits=1  boolean_output=off  mode=Lower Bit Location + Width  bit1=0  base1=MSB of Input  bit0=7  base0=LSB of Input  dbl_ovrd=off  block_type=slice
  b8 : xbsIndex_r4/Slice  nbits=1  boolean_output=off  mode=Lower Bit Location + Width  bit1=0  base1=MSB of Input  bit0=8  base0=LSB of Input  dbl_ovrd=off  block_type=slice
  bool{1..18} (18 alike) : xbsIndex_r4/Convert  gui_display_data_type=Boolean  arith_type=Boolean  n_bits=16  bin_pt=14  float_type=Single  exp_bits=8  fraction_bits=24  quantization=Truncate  overflow=Wrap  en=off  latency=0  dbl_ovrd=off  pipeline=off  block_type=convert
  AND 0 : Outport
  AND 1 : Outport  Port=2
  AND 2 : Outport  Port=3
  AND 3 : Outport  Port=4
  AND 4 : Outport  Port=5
  AND 5 : Outport  Port=6
  AND 6 : Outport  Port=7
  AND 7 : Outport  Port=8
  AND 8 : Outport  Port=9
  OR 0 : Outport  Port=10
  OR 1 : Outport  Port=11
  OR 2 : Outport  Port=12
  OR 3 : Outport  Port=13
  OR 4 : Outport  Port=14
  OR 5 : Outport  Port=15
  OR 6 : Outport  Port=16
  OR 7 : Outport  Port=17
  OR 8 : Outport  Port=18
  wires:
  32b/1 -> b0/1, b1/1, b2/1, b3/1, b4/1, b5/1, b6/1, b7/1, b16/1, b17/1, b18/1, b19/1, b20/1, b21/1, b22/1, b23/1, b24/1, b8/1
  b0/1 -> bool2/1
  b1/1 -> bool1/1
  b2/1 -> bool3/1
  b3/1 -> bool4/1
  b4/1 -> bool5/1
  b5/1 -> bool6/1
  b6/1 -> bool7/1
  b7/1 -> bool8/1
  b16/1 -> bool9/1
  b17/1 -> bool10/1
  b18/1 -> bool11/1
  b19/1 -> bool12/1
  b20/1 -> bool13/1
  b21/1 -> bool14/1
  b22/1 -> bool15/1
  b23/1 -> bool16/1
  bool2/1 -> AND 0/1
  bool1/1 -> AND 1/1
  bool3/1 -> AND 2/1
  bool4/1 -> AND 3/1
  bool5/1 -> AND 4/1
  bool6/1 -> AND 5/1
  bool7/1 -> AND 6/1
  bool8/1 -> AND 7/1
  bool9/1 -> OR 0/1
  bool10/1 -> OR 1/1
  bool11/1 -> OR 2/1
  bool12/1 -> OR 3/1
  bool13/1 -> OR 4/1
  bool14/1 -> OR 5/1
  bool15/1 -> OR 6/1
  bool16/1 -> OR 7/1
  b8/1 -> bool17/1
  bool17/1 -> AND 8/1
  b24/1 -> bool18/1
  bool18/1 -> OR 8/1

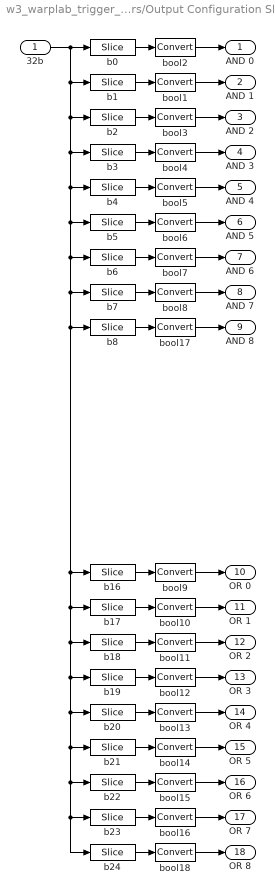
== system w3_warplab_trigger_proc/Registers/Output Configuration Slice9 ==
  32b : Inport
  b0 : xbsIndex_r4/Slice  nbits=1  boolean_output=off  mode=Lower Bit Location + Width  bit1=0  base1=MSB of Input  bit0=0  base0=LSB of Input  dbl_ovrd=off  block_type=slice
  b1 : xbsIndex_r4/Slice  nbits=1  boolean_output=off  mode=Lower Bit Location + Width  bit1=0  base1=MSB of Input  bit0=1  base0=LSB of Input  dbl_ovrd=off  block_type=slice
  b16 : xbsIndex_r4/Slice  nbits=1  boolean_output=off  mode=Lower Bit Location + Width  bit1=0  base1=MSB of Input  bit0=16  base0=LSB of Input  dbl_ovrd=off  block_type=slice
  b17 : xbsIndex_r4/Slice  nbits=1  boolean_output=off  mode=Lower Bit Location + Width  bit1=0  base1=MSB of Input  bit0=17  base0=LSB of Input  dbl_ovrd=off  block_type=slice
  b18 : xbsIndex_r4/Slice  nbits=1  boolean_output=off  mode=Lower Bit Location + Width  bit1=0  base1=MSB of Input  bit0=18  base0=LSB of Input  dbl_ovrd=off  block_type=slice
  b19 : xbsIndex_r4/Slice  nbits=1  boolean_output=off  mode=Lower Bit Location + Width  bit1=0  base1=MSB of Input  bit0=19  base0=LSB of Input  dbl_ovrd=off  block_type=slice
  b2 : xbsIndex_r4/Slice  nbits=1  boolean_output=off  mode=Lower Bit Location + Width  bit1=0  base1=MSB of Input  bit0=2  base0=LSB of Input  dbl_ovrd=off  block_type=slice
  b20 : xbsIndex_r4/Slice  nbits=1  boolean_output=off  mode=Lower Bit Location + Width  bit1=0  base1=MSB of Input  bit0=20  base0=LSB of Input  dbl_ovrd=off  block_type=slice
  b21 : xbsIndex_r4/Slice  nbits=1  boolean_output=off  mode=Lower Bit Location + Width  bit1=0  base1=MSB of Input  bit0=21  base0=LSB of Input  dbl_ovrd=off  block_type=slice
  b22 : xbsIndex_r4/Slice  nbits=1  boolean_output=off  mode=Lower Bit Location + Width  bit1=0  base1=MSB of Input  bit0=22  base0=LSB of Input  dbl_ovrd=off  block_type=slice
  b23 : xbsIndex_r4/Slice  nbits=1  boolean_output=off  mode=Lower Bit Location + Width  bit1=0  base1=MSB of Input  bit0=23  base0=LSB of Input  dbl_ovrd=off  block_type=slice
  b24 : xbsIndex_r4/Slice  nbits=1  boolean_output=off  mode=Lower Bit Location + Width  bit1=0  base1=MSB of Input  bit0=24  base0=LSB of Input  dbl_ovrd=off  block_type=slice
  b3 : xbsIndex_r4/Slice  nbits=1  boolean_output=off  mode=Lower Bit Location + Width  bit1=0  base1=MSB of Input  bit0=3  base0=LSB of Input  dbl_ovrd=off  block_type=slice
  b4 : xbsIndex_r4/Slice  nbits=1  boolean_output=off  mode=Lower Bit Location + Width  bit1=0  base1=MSB of Input  bit0=4  base0=LSB of Input  dbl_ovrd=off  block_type=slice
  b5 : xbsIndex_r4/Slice  nbits=1  boolean_output=off  mode=Lower Bit Location + Width  bit1=0  base1=MSB of Input  bit0=5  base0=LSB of Input  dbl_ovrd=off  block_type=slice
  b6 : xbsIndex_r4/Slice  nbits=1  boolean_output=off  mode=Lower Bit Location + Width  bit1=0  base1=MSB of Input  bit0=6  base0=LSB of Input  dbl_ovrd=off  block_type=slice
  b7 : xbsIndex_r4/Slice  nbits=1  boolean_output=off  mode=Lower Bit Location + Width  bit1=0  base1=MSB of Input  bit0=7  base0=LSB of Input  dbl_ovrd=off  block_type=slice
  b8 : xbsIndex_r4/Slice  nbits=1  boolean_output=off  mode=Lower Bit Location + Width  bit1=0  base1=MSB of Input  bit0=8  base0=LSB of Input  dbl_ovrd=off  block_type=slice
  bool{1..18} (18 alike) : xbsIndex_r4/Convert  gui_display_data_type=Boolean  arith_type=Boolean  n_bits=16  bin_pt=14  float_type=Single  exp_bits=8  fraction_bits=24  quantization=Truncate  overflow=Wrap  en=off  latency=0  dbl_ovrd=off  pipeline=off  block_type=convert
  AND 0 : Outport
  AND 1 : Outport  Port=2
  AND 2 : Outport  Port=3
  AND 3 : Outport  Port=4
  AND 4 : Outport  Port=5
  AND 5 : Outport  Port=6
  AND 6 : Outport  Port=7
  AND 7 : Outport  Port=8
  AND 8 : Outport  Port=9
  OR 0 : Outport  Port=10
  OR 1 : Outport  Port=11
  OR 2 : Outport  Port=12
  OR 3 : Outport  Port=13
  OR 4 : Outport  Port=14
  OR 5 : Outport  Port=15
  OR 6 : Outport  Port=16
  OR 7 : Outport  Port=17
  OR 8 : Outport  Port=18
  wires:
  32b/1 -> b0/1, b1/1, b2/1, b3/1, b4/1, b5/1, b6/1, b7/1, b16/1, b17/1, b18/1, b19/1, b20/1, b21/1, b22/1, b23/1, b24/1, b8/1
  b0/1 -> bool2/1
  b1/1 -> bool1/1
  b2/1 -> bool3/1
  b3/1 -> bool4/1
  b4/1 -> bool5/1
  b5/1 -> bool6/1
  b6/1 -> bool7/1
  b7/1 -> bool8/1
  b16/1 -> bool9/1
  b17/1 -> bool10/1
  b18/1 -> bool11/1
  b19/1 -> bool12/1
  b20/1 -> bool13/1
  b21/1 -> bool14/1
  b22/1 -> bool15/1
  b23/1 -> bool16/1
  bool2/1 -> AND 0/1
  bool1/1 -> AND 1/1
  bool3/1 -> AND 2/1
  bool4/1 -> AND 3/1
  bool5/1 -> AND 4/1
  bool6/1 -> AND 5/1
  bool7/1 -> AND 6/1
  bool8/1 -> AND 7/1
  bool9/1 -> OR 0/1
  bool10/1 -> OR 1/1
  bool11/1 -> OR 2/1
  bool12/1 -> OR 3/1
  bool13/1 -> OR 4/1
  bool14/1 -> OR 5/1
  bool15/1 -> OR 6/1
  bool16/1 -> OR 7/1
  b8/1 -> bool17/1
  bool17/1 -> AND 8/1
  b24/1 -> bool18/1
  bool18/1 -> OR 8/1

== system w3_warplab_trigger_proc/Registers/Trig IODELAY Config ==
  From Register1 : xbsIndex_r4/From Register  shared_memory_name='TRIG_IODELAYS_CONTROL'  init=0  period=1  ownership=Locally owned and initialized  gui_display_data_type=Fixed-point  arith_type=Unsigned  n_bits=32  bin_pt=0  preci_type=Single  dbl_ovrd=off  block_type=fromreg
      settings: AttributesFormatString=<< %<shared_memory_name> >>  infoedit="Register block that reads data to a shared memory register.  Delay of one sample period."  block_version=8.2
  From Register25 : xbsIndex_r4/From Register  shared_memory_name='TRIG_IDELAY_CFG_DEBUG_HDR'  init=0  period=1  ownership=Locally owned and initialized  gui_display_data_type=Fixed-point  arith_type=Unsigned  n_bits=32  bin_pt=0  preci_type=Single  dbl_ovrd=off  block_type=fromreg
      settings: AttributesFormatString=<< %<shared_memory_name> >>  infoedit="Register block that reads data to a shared memory register.  Delay of one sample period."  block_version=8.2
  From Register26 : xbsIndex_r4/From Register  shared_memory_name='TRIG_ODELAY_CFG_DEBUG_HDR'  init=0  period=1  ownership=Locally owned and initialized  gui_display_data_type=Fixed-point  arith_type=Unsigned  n_bits=32  bin_pt=0  preci_type=Single  dbl_ovrd=off  block_type=fromreg
      settings: AttributesFormatString=<< %<shared_memory_name> >>  infoedit="Register block that reads data to a shared memory register.  Delay of one sample period."  block_version=8.2
  From Register27 : xbsIndex_r4/From Register  shared_memory_name='TRIG_IDELAY_CFG_CMPLL'  init=0  period=1  ownership=Locally owned and initialized  gui_display_data_type=Fixed-point  arith_type=Unsigned  n_bits=32  bin_pt=0  preci_type=Single  dbl_ovrd=off  block_type=fromreg
      settings: AttributesFormatString=<< %<shared_memory_name> >>  infoedit="Register block that reads data to a shared memory register.  Delay of one sample period."  block_version=8.2
  From Register28 : xbsIndex_r4/From Register  shared_memory_name='TRIG_ODELAY_CFG_CMPLL'  init=0  period=1  ownership=Locally owned and initialized  gui_display_data_type=Fixed-point  arith_type=Unsigned  n_bits=32  bin_pt=0  preci_type=Single  dbl_ovrd=off  block_type=fromreg
      settings: AttributesFormatString=<< %<shared_memory_name> >>  infoedit="Register block that reads data to a shared memory register.  Delay of one sample period."  block_version=8.2
  b[0] : xbsIndex_r4/Slice  nbits=1  boolean_output=off  mode=Lower Bit Location + Width  bit1=0  base1=MSB of Input  bit0=0  base0=LSB of Input  dbl_ovrd=off  block_type=slice
  b[12:8]{,1..3} (4 alike) : xbsIndex_r4/Slice  nbits=5  boolean_output=off  mode=Lower Bit Location + Width  bit1=0  base1=MSB of Input  bit0=8  base0=LSB of Input  dbl_ovrd=off  block_type=slice
  b[1] : xbsIndex_r4/Slice  nbits=1  boolean_output=off  mode=Lower Bit Location + Width  bit1=0  base1=MSB of Input  bit0=1  base0=LSB of Input  dbl_ovrd=off  block_type=slice
  b[20:16]{,1..3} (4 alike) : xbsIndex_r4/Slice  nbits=5  boolean_output=off  mode=Lower Bit Location + Width  bit1=0  base1=MSB of Input  bit0=16  base0=LSB of Input  dbl_ovrd=off  block_type=slice
  b[28:24]{,1..3} (4 alike) : xbsIndex_r4/Slice  nbits=5  boolean_output=off  mode=Lower Bit Location + Width  bit1=0  base1=MSB of Input  bit0=24  base0=LSB of Input  dbl_ovrd=off  block_type=slice
  b[4:0]{,1..3} (4 alike) : xbsIndex_r4/Slice  nbits=5  boolean_output=off  mode=Lower Bit Location + Width  bit1=0  base1=MSB of Input  bit0=0  base0=LSB of Input  dbl_ovrd=off  block_type=slice
  tag scope: TRIG_IN_IDELAYS_UPDATE=global, TRIG_IN_IDELAY_CMPLL0=global, TRIG_IN_IDELAY_CMPLL1=global, TRIG_IN_IDELAY_CMPLL2=global, TRIG_IN_IDELAY_CMPLL3=global, TRIG_IN_IDELAY_DBG0=global, TRIG_IN_IDELAY_DBG1=global, TRIG_IN_IDELAY_DBG2=global, TRIG_IN_IDELAY_DBG3=global, TRIG_OUT_ODELAYS_UPDATE=global, TRIG_OUT_ODELAY_CMPLL0=global, TRIG_OUT_ODELAY_CMPLL1=global, TRIG_OUT_ODELAY_CMPLL2=global, TRIG_OUT_ODELAY_CMPLL3=global, TRIG_OUT_ODELAY_DBG0=global, TRIG_OUT_ODELAY_DBG1=global, TRIG_OUT_ODELAY_DBG2=global, TRIG_OUT_ODELAY_DBG3=global
  wires:
  From Register25/1 -> b[4:0]/1, b[12:8]/1, b[20:16]/1, b[28:24]/1
  b[4:0]/1 -> [TRIG_IN_IDELAY_DBG0]
  b[12:8]/1 -> [TRIG_IN_IDELAY_DBG1]
  b[20:16]/1 -> [TRIG_IN_IDELAY_DBG2]
  b[28:24]/1 -> [TRIG_IN_IDELAY_DBG3]
  b[4:0]1/1 -> [TRIG_OUT_ODELAY_DBG0]
  b[12:8]1/1 -> [TRIG_OUT_ODELAY_DBG1]
  b[20:16]1/1 -> [TRIG_OUT_ODELAY_DBG2]
  b[28:24]1/1 -> [TRIG_OUT_ODELAY_DBG3]
  From Register26/1 -> b[4:0]1/1, b[12:8]1/1, b[20:16]1/1, b[28:24]1/1
  b[4:0]2/1 -> [TRIG_IN_IDELAY_CMPLL0]
  b[12:8]2/1 -> [TRIG_IN_IDELAY_CMPLL1]
  b[20:16]2/1 -> [TRIG_IN_IDELAY_CMPLL2]
  b[28:24]2/1 -> [TRIG_IN_IDELAY_CMPLL3]
  From Register27/1 -> b[4:0]2/1, b[12:8]2/1, b[20:16]2/1, b[28:24]2/1
  b[4:0]3/1 -> [TRIG_OUT_ODELAY_CMPLL0]
  b[12:8]3/1 -> [TRIG_OUT_ODELAY_CMPLL1]
  b[20:16]3/1 -> [TRIG_OUT_ODELAY_CMPLL2]
  b[28:24]3/1 -> [TRIG_OUT_ODELAY_CMPLL3]
  From Register28/1 -> b[4:0]3/1, b[12:8]3/1, b[20:16]3/1, b[28:24]3/1
  From Register1/1 -> b[0]/1, b[1]/1
  b[0]/1 -> [TRIG_IN_IDELAYS_UPDATE]
  b[1]/1 -> [TRIG_OUT_ODELAYS_UPDATE]

== system w3_warplab_trigger_proc/Trigger Sources/AGC ==
  Constant2 : Constant  Value=0
  agc_done_in : xbsIndex_r4/Gateway In  gui_display_data_type=Fixed-point  arith_type=Unsigned  n_bits=1  bin_pt=0  preci_type=Single  exp_width=8  frac_width=24  quantization="Round  (unbiased: +/- Inf)"  overflow=Wrap  period=1  dbl_ovrd=off  timing_constraint=None  locs_specified=off  LOCs={}  UseAsADC=off  ADCChannel='1'  inherit_from_input=off  hdl_port=on  block_type=gatewayin
  Trigger : Outport
  wires:
  agc_done_in/1 -> Trigger/1
  Constant2/1 -> agc_done_in/1

== system w3_warplab_trigger_proc/Trigger Sources/Align ==
  D : Inport
  Down Sample3 : xbsIndex_r4/Down Sample  sample_ratio=4  sample_phase="Last Value of Frame  (most efficient)"  en=off  latency=1  dbl_ovrd=off  block_type=dsamp
  Up Sample : xbsIndex_r4/Up Sample  sample_ratio=4  copy_samples=on  en=off  latency=0  dbl_ovrd=off  block_type=usamp
  Q : Outport
  wires:
  Down Sample3/1 -> Up Sample/1
  D/1 -> Down Sample3/1
  Up Sample/1 -> Q/1

== system w3_warplab_trigger_proc/Trigger Sources/Align1 ==
  D : Inport
  Down Sample3 : xbsIndex_r4/Down Sample  sample_ratio=4  sample_phase="Last Value of Frame  (most efficient)"  en=off  latency=1  dbl_ovrd=off  block_type=dsamp
  Up Sample : xbsIndex_r4/Up Sample  sample_ratio=4  copy_samples=on  en=off  latency=0  dbl_ovrd=off  block_type=usamp
  Q : Outport
  wires:
  Up Sample/1 -> Q/1
  D/1 -> Down Sample3/1
  Down Sample3/1 -> Up Sample/1

== system w3_warplab_trigger_proc/Trigger Sources/Align2 ==
  D : Inport
  Down Sample3 : xbsIndex_r4/Down Sample  sample_ratio=4  sample_phase="Last Value of Frame  (most efficient)"  en=off  latency=1  dbl_ovrd=off  block_type=dsamp
  Up Sample : xbsIndex_r4/Up Sample  sample_ratio=4  copy_samples=on  en=off  latency=0  dbl_ovrd=off  block_type=usamp
  Q : Outport
  wires:
  Down Sample3/1 -> Up Sample/1
  D/1 -> Down Sample3/1
  Up Sample/1 -> Q/1

== system w3_warplab_trigger_proc/Trigger Sources/Align3 ==
  D : Inport
  Down Sample3 : xbsIndex_r4/Down Sample  sample_ratio=4  sample_phase="Last Value of Frame  (most efficient)"  en=off  latency=1  dbl_ovrd=off  block_type=dsamp
  Up Sample : xbsIndex_r4/Up Sample  sample_ratio=4  copy_samples=on  en=off  latency=0  dbl_ovrd=off  block_type=usamp
  Q : Outport
  wires:
  Up Sample/1 -> Q/1
  D/1 -> Down Sample3/1
  Down Sample3/1 -> Up Sample/1

== system w3_warplab_trigger_proc/Trigger Sources/Align8 ==
  D : Inport
  Down Sample3 : xbsIndex_r4/Down Sample  sample_ratio=4  sample_phase="Last Value of Frame  (most efficient)"  en=off  latency=1  dbl_ovrd=off  block_type=dsamp
  Up Sample : xbsIndex_r4/Up Sample  sample_ratio=4  copy_samples=on  en=off  latency=0  dbl_ovrd=off  block_type=usamp
  Q : Outport
  wires:
  Down Sample3/1 -> Up Sample/1
  D/1 -> Down Sample3/1
  Up Sample/1 -> Q/1

== system w3_warplab_trigger_proc/Trigger Sources/CM PLL 0 ==
  " Debounce Register1" : xbsIndex_r4/Register  init=0  rst=off  en=off  dbl_ovrd=off  block_type=register
  Debounce Register2 : xbsIndex_r4/Register  init=0  rst=off  en=off  dbl_ovrd=off  block_type=register
  Debounce Register3 : xbsIndex_r4/Register  init=0  rst=off  en=off  dbl_ovrd=off  block_type=register
  Debounce Register4 : xbsIndex_r4/Register  init=0  rst=off  en=off  dbl_ovrd=off  block_type=register
  Logical : xbsIndex_r4/Logical  logical_function=AND  inputs=4  en=off  latency=0  precision=Full  arith_type=Unsigned  n_bits=16  bin_pt=0  align_bp=on  dbl_ovrd=off  block_type=logical
  Mux : xbsIndex_r4/Mux  inputs=2  en=off  latency=0  precision=Full  arith_type=Unsigned  n_bits=16  bin_pt=14  quantization=Truncate  overflow=Wrap  dbl_ovrd=off  block_type=mux
  Trigger : Outport
  wires:
  Mux/1 -> Trigger/1
  [TRIG_DELAYED_CM_PLL_0] -> Mux/2, " Debounce Register1"/1
  " Debounce Register1"/1 -> Debounce Register2/1, Logical/1
  Debounce Register2/1 -> Logical/2, Debounce Register3/1
  Debounce Register3/1 -> Debounce Register4/1, Logical/3
  [Debug_0_Debounce] -> Mux/1
  Debounce Register4/1 -> Logical/4
  Logical/1 -> Mux/3

== system w3_warplab_trigger_proc/Trigger Sources/CM PLL 1 ==
  Debounce Register{1..4} (4 alike) : xbsIndex_r4/Register  init=0  rst=off  en=off  dbl_ovrd=off  block_type=register
  Logical : xbsIndex_r4/Logical  logical_function=AND  inputs=4  en=off  latency=0  precision=Full  arith_type=Unsigned  n_bits=16  bin_pt=0  align_bp=on  dbl_ovrd=off  block_type=logical
  Mux : xbsIndex_r4/Mux  inputs=2  en=off  latency=0  precision=Full  arith_type=Unsigned  n_bits=16  bin_pt=14  quantization=Truncate  overflow=Wrap  dbl_ovrd=off  block_type=mux
  Trigger : Outport
  wires:
  Logical/1 -> Mux/3
  Debounce Register4/1 -> Logical/4
  [Debug_1_Debounce] -> Mux/1
  Debounce Register3/1 -> Logical/3, Debounce Register4/1
  Debounce Register2/1 -> Logical/2, Debounce Register3/1
  Debounce Register1/1 -> Logical/1, Debounce Register2/1
  Mux/1 -> Trigger/1
  [TRIG_DELAYED_CM_PLL_1] -> Debounce Register1/1, Mux/2
